simulink model "mpc555rt_led"  (Simulink 6.0)
settings: Solver=FixedStepDiscrete  StartTime=0.0  StopTime=inf  FixedStep=0.01  RelTol=1e-3
PreLoadFcn:
  | RTWConfigurationCB('preloadfcn', bdroot);
libraries: mpc555drivers x2
CloseFcn:
  | rtwprivate ssgencode ModelCloseRequest foo
settings Model: Creator=The MathWorks Inc.  LastModifiedBy=batserve  ExtModeAutoUpdateStatusClock=off  ProdHWDeviceType=Motorola PowerPC
settings DataIOCC: SignalLoggingName=sigsOut
settings OptimizationCC: BooleanDataType=off  InlineParams=on  InlineInvariantSignals=off  OptimizeModelRefInitCode=on  LifeSpan=1
settings DebuggingCC: CheckExecutionContextPreStartOutputMsg=on  CheckExecutionContextRuntimeOutputMsg=on  SolverPrmCheckMsg=none
settings HardwareCC: ProdEndianess=BigEndian  ProdHWDeviceType=Motorola PowerPC
settings RTWCC: SystemTargetFile=mpc555rt.tlc  TemplateMakefile=mpc555rt.tmf  ProcessScript=mpc555rt_make_rtw_hook
settings CodeAppCC: IgnoreCustomStorageClasses=off
settings STFCustomTargetCC: TargetFcnLib=ansi_tfl_tmw.mat  GenFloatMathFcnCalls=ANSI_C  ModelReferenceCompliant=off  CombineOutputUpdateFcns=on  ERTCustomFileBanners=on  SystemTargetFile=mpc555rt.tlc
settings ERTTargetCC: TargetFcnLib=ansi_tfl_tmw.mat  GenFloatMathFcnCalls=ANSI_C  ModelReferenceCompliant=off  SupportContinuousTime=on  SupportNonInlinedSFcns=on  RootIOFormat=Individual Arguments  ERTCustomFileTemplate=example_file_process.tlc  InitialValueSource=Model
settings CustomProperty: DataType=RTWOptions_EnumType__toolbox_rtw_targets_mpc555dk_mpc555dk_mpc555rt_MPC555_OPTIMIZATION_SWITCH  Value=speed
settings EnumStrPairs: String=speed

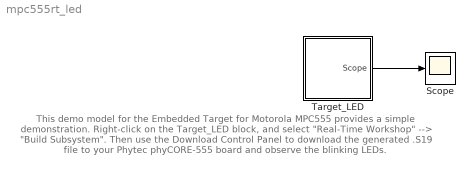
== system mpc555rt_led ==
  note: This demo model for the Embedded Target for
      | Motorola MPC555 provides a simple demonstration.
      |
      | Right-click on the Target_LED block, and select
      | "Real-Time Workshop" --> "Build Subsystem".
      | Then use the Download Control Panel to
      | download the generated .S19 file to your
      | Phytec phyCORE-555 board and observe the
      | blinking LEDs.
  Scope : Scope
      settings: YMin=0  YMax=1
  Target_LED : Subsystem  InitFcn=|  PropExecContextAcrossSSBoundary=on
      | % START RTW CONFIGURATION CODE %
      | RTWConfigurationCB('rtw_target_initfcn',gcb);
      | % END RTW CONFIGURATION CODE %
      mask Display: image(imread('target_affordance_icon.jpg'),'bottom-right')
  wires:
  Target_LED/1(Scope) -> Scope/1

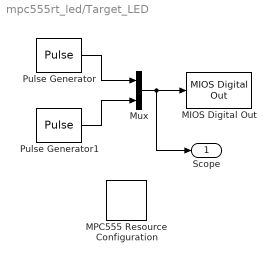
== system mpc555rt_led/Target_LED ==
  MIOS Digital Out : mpc555drivers/Modular Input//Output System (MIOS1)/MIOS Digital Out  bits=[0 1]  t=-1  enablePassThru=off
  MPC555 Resource Configuration : mpc555drivers/MPC555 Resource Configuration  Tag=RTW CONFIGURATION BLOCK  AncestorBlock=|  oldParentName=mpc555rt_led/Target_LED  oldBlockName=|  defaultConfigLibrary=mpc555drivers
      AncestorBlock=|
      | config_library/Subsystem
      | Resource
      | Configuration
      oldBlockName=|
      | mpc555rt_led/Target_LED/MPC555
      | Resource
      | Configuration
  Mux : Mux  Inputs=2
  Pulse Generator : DiscretePulseGenerator  Period=100  PulseWidth=50  SampleTime=0.01  VectorParams1D=off
  Pulse Generator1 : DiscretePulseGenerator  Period=50  PulseWidth=25  SampleTime=0.01
  Scope : Outport
  wires:
  Mux/1 -> MIOS Digital Out/1, Scope/1
  Pulse Generator/1 -> Mux/1
  Pulse Generator1/1 -> Mux/2
